simulink model "sampleModel1"  (R2021a)
settings: Solver=VariableStepAuto  StartTime=0.0  StopTime=50  RelTol=1e-3
undefined symbols (not defined in the file): DiscIntNeverNeededParam, magnitude, Newton, Raphson
libraries: simulink x92, pid_lib x10
(part 3 of 5)

== system sampleModel1/cfblk104/cfblk19/cfblk13 ==
  cfblk1 : Inport
  cfblk10 : Inport  Port=2
  cfblk3 : simulink/Discrete/Transfer Fcn Real Zero  ZeroZ=0.75  ICPrevInput=0.0  DoSatur=off
      settings: SourceProductBaseCode=SL
  cfblk4 : Product  Inputs=*
  cfblk5 : Sum  Inputs=+
  cfblk6 : Constant  Value=[-896346582.191985]  SampleTime=1
  cfblk7 : Constant  Value=[-330190841.244627]  SampleTime=1
  cfblk8 : Constant  Value=[644803615.291474]  SampleTime=1
  cfblk9 : Constant  Value=[-669058809.263533]  SampleTime=1
  cfblk2 : Outport
  cfblk11 : Outport  Port=2
  wires:
  cfblk8/1 -> cfblk11/1
  cfblk10/1 -> cfblk5/1
  cfblk9/1 -> cfblk4/1
  cfblk7/1 -> cfblk2/1
  cfblk4/1 -> cfblk3/1

== system sampleModel1/cfblk104/cfblk19/cfblk17 ==
  cfblk1 : Inport
  cfblk15 : Inport  Port=2
  Action Port : ActionPort  ActionPortLabel=if(u1 >= 0)
  cfblk10 : Constant  Value=[-692720338.214887]  SampleTime=1
  cfblk11 : Constant  Value=[-981830203.016373]  SampleTime=1
  cfblk12 : Subsystem
  cfblk13 : Subsystem
  cfblk14 : If  IfExpression=u1 >= 0  SampleTime=1
  cfblk16 : Subsystem  TreatAsAtomicUnit=on
  cfblk17 : Subsystem  TreatAsAtomicUnit=on
  cfblk18 : Delay
  cfblk3 : DiscreteFir
  cfblk4 : UnaryMinus
  cfblk5 : Signum
  cfblk6 : Product  Inputs=**
  cfblk7 : Constant  Value=[115715381.439592]  SampleTime=1
  cfblk8 : Constant  Value=[789801584.459016]  SampleTime=1
  cfblk9 : Constant  Value=[-738286634.708104]  SampleTime=1
  cfblk2 : Outport
  wires:
  cfblk10/1 -> cfblk6/1
  cfblk4/1 -> cfblk17/1(cfblk1)
  cfblk12/1(cfblk2) -> cfblk3/1
  cfblk17/1(cfblk2) -> cfblk2/1
  cfblk11/1 -> cfblk5/1, cfblk12/6(cfblk12)
  cfblk13/1(cfblk2) -> cfblk16/1(cfblk1)
  cfblk12/2(cfblk13) -> cfblk13/1(cfblk1)
  cfblk16/1(cfblk2) -> cfblk17/2(cfblk9)
  cfblk8/1 -> cfblk6/2
  cfblk3/1 -> cfblk16/2(cfblk7)
  cfblk7/1 -> cfblk14/1
  cfblk5/1 -> cfblk12/1(cfblk1)
  cfblk6/1 -> cfblk4/1
  cfblk9/1 -> cfblk12/2(cfblk8)
  cfblk15/1 -> cfblk12/3(cfblk9)
  cfblk1/1 -> cfblk12/4(cfblk10)
  cfblk14/1 -> cfblk16/Action
  cfblk14/2 -> cfblk17/Action
  cfblk13/2(cfblk14) -> cfblk18/1
  cfblk18/1 -> cfblk12/5(cfblk11)

== system sampleModel1/cfblk104/cfblk19/cfblk18 ==
  cfblk1 : Inport
  cfblk8 : Inport  Port=2
  Action Port : ActionPort  ActionPortLabel=else
  cfblk11 : Delay
  cfblk3 : Sqrt  Operator=rSqrt  AlgorithmType=Newton-Raphson  SaturateOnIntegerOverflow=on
  cfblk4 : Sqrt  SaturateOnIntegerOverflow=on
  cfblk5 : ComplexToRealImag
  cfblk6 : Constant  Value=[-692674466.938590]  SampleTime=1
  cfblk7 : Subsystem
  cfblk2 : Outport
  cfblk9 : Outport  Port=2
  cfblk10 : Outport  Port=3
  wires:
  cfblk5/1 -> cfblk10/1
  cfblk4/1 -> cfblk7/1(cfblk1), cfblk9/1
  cfblk8/1 -> cfblk7/2(cfblk9)
  cfblk6/1 -> cfblk4/1
  cfblk1/1 -> cfblk2/1
  cfblk3/1 -> cfblk7/3(cfblk10)
  cfblk7/1(cfblk2) -> cfblk5/1
  cfblk5/2 -> cfblk11/1
  cfblk11/1 -> cfblk3/1

== system sampleModel1/cfblk104/cfblk21/cfblk11 ==
  cfblk1 : Inport
  cfblk13 : Inport  Port=2
  Action Port : ActionPort  ActionPortLabel=if(u1 >= 0)
  cfblk10 : Constant  Value=[-563913250.111774]  SampleTime=1
  cfblk11 : Subsystem
  cfblk12 : Subsystem
  cfblk16 : Delay
  cfblk3 : DiscreteFir
  cfblk4 : Math  Operator=conj  SaturateOnIntegerOverflow=on
  cfblk5 : Gain  Gain=[532058728.474376]
  cfblk6 : Trigonometry
  cfblk7 : simulink/Math Operations/Slider Gain  gain=1  low=0  high=2
  cfblk8 : Constant  Value=[692304688.549677]  SampleTime=1
  cfblk9 : Constant  Value=[191414295.157756]  SampleTime=1
  cfblk2 : Outport
  cfblk14 : Outport  Port=2
  cfblk15 : Outport  Port=3
  wires:
  cfblk9/1 -> cfblk4/1
  cfblk11/1(cfblk2) -> cfblk7/1
  cfblk10/1 -> cfblk14/1
  cfblk3/1 -> cfblk15/1
  cfblk1/1 -> cfblk12/1(cfblk1)
  cfblk4/1 -> cfblk3/1
  cfblk13/1 -> cfblk6/1
  cfblk6/1 -> cfblk5/1
  cfblk8/1 -> cfblk11/1(cfblk1)
  cfblk5/1 -> cfblk2/1
  cfblk12/1(cfblk2) -> cfblk11/2(cfblk10)
  cfblk7/1 -> cfblk16/1
  cfblk16/1 -> cfblk11/3(cfblk11)

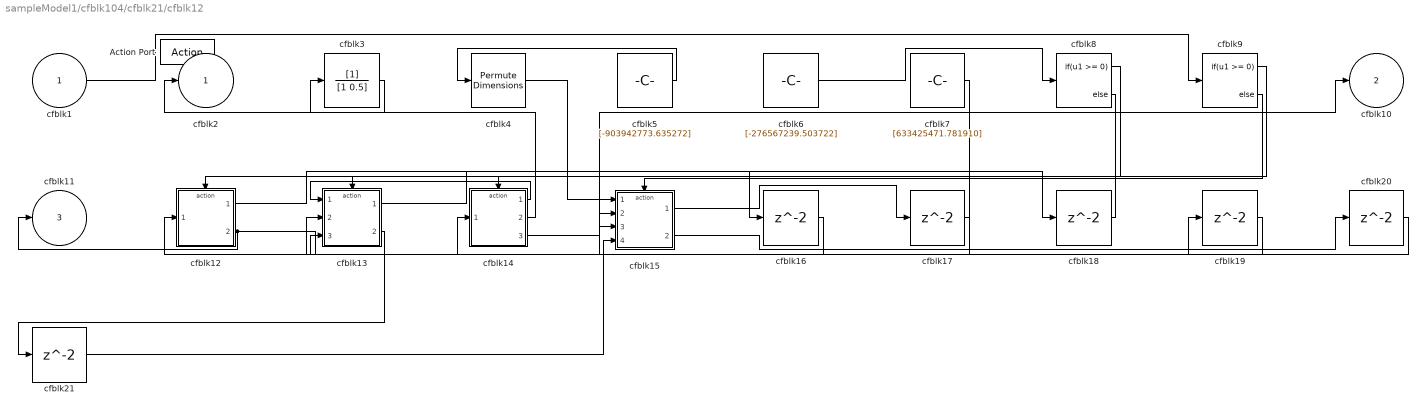
== system sampleModel1/cfblk104/cfblk21/cfblk12 ==
  cfblk1 : Inport
  Action Port : ActionPort  ActionPortLabel=else
  cfblk12 : Subsystem  TreatAsAtomicUnit=on
  cfblk13 : Subsystem  TreatAsAtomicUnit=on
  cfblk14 : Subsystem  TreatAsAtomicUnit=on
  cfblk15 : Subsystem  TreatAsAtomicUnit=on
  cfblk{16..21} (6 alike) : Delay
  cfblk3 : DiscreteFilter
  cfblk4 : PermuteDimensions
  cfblk5 : Constant  Value=[-903942773.635272]  SampleTime=1
  cfblk6 : Constant  Value=[-276567239.503722]  SampleTime=1
  cfblk7 : Constant  Value=[633425471.781910]  SampleTime=1
  cfblk8 : If  IfExpression=u1 >= 0  SampleTime=1
  cfblk9 : If  IfExpression=u1 >= 0  SampleTime=1
  cfblk2 : Outport
  cfblk10 : Outport  Port=2
  cfblk11 : Outport  Port=3
  wires:
  cfblk3/1 -> cfblk2/1
  cfblk5/1 -> cfblk4/1
  cfblk4/1 -> cfblk15/1(cfblk1)
  cfblk7/1 -> cfblk14/1(cfblk1)
  cfblk6/1 -> cfblk8/1
  cfblk12/2(cfblk10) -> cfblk11/1, cfblk19/1
  cfblk1/1 -> cfblk9/1
  cfblk14/1(cfblk2) -> cfblk13/1(cfblk1)
  cfblk14/2(cfblk14) -> cfblk3/1
  cfblk14/3(cfblk15) -> cfblk10/1
  cfblk8/1 -> cfblk12/Action
  cfblk8/2 -> cfblk13/Action
  cfblk9/1 -> cfblk14/Action
  cfblk9/2 -> cfblk15/Action
  cfblk13/1(cfblk2) -> cfblk16/1
  cfblk16/1 -> cfblk15/3(cfblk14)
  cfblk15/1(cfblk2) -> cfblk17/1
  cfblk17/1 -> cfblk12/1(cfblk1)
  cfblk12/1(cfblk2) -> cfblk18/1
  cfblk18/1 -> cfblk15/2(cfblk13)
  cfblk19/1 -> cfblk13/3(cfblk7)
  cfblk15/2(cfblk16) -> cfblk20/1
  cfblk20/1 -> cfblk13/2(cfblk6)
  cfblk13/2(cfblk8) -> cfblk21/1
  cfblk21/1 -> cfblk15/4(cfblk15)

== system sampleModel1/cfblk105/cfblk6/cfblk10 ==
  cfblk1 : Inport
  cfblk12 : Inport  Port=2
  Action Port : ActionPort  ActionPortLabel=else
  cfblk10 : Subsystem
  cfblk11 : If  IfExpression=u1 >= 0  SampleTime=1
  cfblk14 : Subsystem  TreatAsAtomicUnit=on
  cfblk15 : Subsystem  TreatAsAtomicUnit=on
  cfblk16 : Delay
  cfblk17 : Delay
  cfblk18 : Delay
  cfblk3 : ComplexToMagnitudeAngle
  cfblk4 : MinMax  Function=max
  cfblk5 : Trigonometry
  cfblk6 : Product
  cfblk7 : Constant  Value=[986074348.650515]  SampleTime=1
  cfblk8 : Constant  Value=[-373705013.156286]  SampleTime=1
  cfblk9 : Constant  Value=[204800515.931455]  SampleTime=1
  cfblk2 : Outport
  cfblk13 : Outport  Port=2
  wires:
  cfblk6/1 -> cfblk5/1
  cfblk5/1 -> cfblk15/1(cfblk1)
  cfblk9/1 -> cfblk6/1
  cfblk3/1 -> cfblk2/1
  cfblk10/1(cfblk2) -> cfblk13/1
  cfblk14/1(cfblk2) -> cfblk4/1
  cfblk8/1 -> cfblk10/1(cfblk1)
  cfblk10/2(cfblk10) -> cfblk3/1
  cfblk7/1 -> cfblk6/2
  cfblk12/1 -> cfblk14/1(cfblk1)
  cfblk14/2(cfblk15) -> cfblk10/2(cfblk9)
  cfblk14/3(cfblk16) -> cfblk15/2(cfblk9)
  cfblk1/1 -> cfblk14/4(cfblk14)
  cfblk11/1 -> cfblk14/Action
  cfblk11/2 -> cfblk15/Action
  cfblk4/1 -> cfblk16/1
  cfblk16/1 -> cfblk14/2(cfblk12)
  cfblk3/2 -> cfblk17/1
  cfblk17/1 -> cfblk11/1
  cfblk15/1(cfblk2) -> cfblk18/1
  cfblk18/1 -> cfblk14/3(cfblk13)

== system sampleModel1/cfblk105/cfblk6/cfblk9 ==
  cfblk1 : Inport
  cfblk8 : Inport  Port=2
  Action Port : ActionPort  ActionPortLabel=if(u1 >= 0)
  cfblk3 : MinMax  Function=max  Inputs=2
  cfblk4 : simulink/Math Operations/Slider Gain  gain=1  low=0  high=2
  cfblk5 : Polyval  Coefs=[ +2.081618890e-019, -1.441693666e-014, +4.719686976e-010, -8.536869453e-006, +1.621573104e-001, -8.087801117e+001 ]
  cfblk6 : Product  Inputs=**
  cfblk7 : Constant  Value=[-112981505.131855]  SampleTime=1
  cfblk2 : Outport
  wires:
  cfblk5/1 -> cfblk2/1
  cfblk1/1 -> cfblk6/1
  cfblk4/1 -> cfblk3/1
  cfblk3/1 -> cfblk5/1
  cfblk8/1 -> cfblk3/2
  cfblk7/1 -> cfblk6/2
  cfblk6/1 -> cfblk4/1

== system sampleModel1/cfblk108/cfblk9/cfblk7 ==
  cfblk1 : Inport
  cfblk11 : Delay
  cfblk3 : simulink/Discrete/Tapped Delay  vinit=0.0  samptime=-1  NumDelays=1  DelayOrder=Oldest  includeCurrent=off
  cfblk4 : Sum  Inputs=-+
  cfblk5 : Assignment  DiagnosticForDimensions=Warning  IndexOptions=Index vector (dialog)  Indices=1  OutputSizes=1
  cfblk6 : Trigonometry
  cfblk7 : Constant  Value=[85798913.173892]  SampleTime=1
  cfblk8 : Constant  Value=[43764762.818563]  SampleTime=1
  cfblk9 : Constant  Value=[-705776039.354427]  SampleTime=1
  cfblk2 : Outport
  cfblk10 : Outport  Port=2
  wires:
  cfblk7/1 -> cfblk3/1
  cfblk1/1 -> cfblk2/1
  cfblk3/1 -> cfblk5/1
  cfblk9/1 -> cfblk4/2
  cfblk4/1 -> cfblk6/1
  cfblk8/1 -> cfblk5/2
  cfblk5/1 -> cfblk10/1
  cfblk6/1 -> cfblk11/1
  cfblk11/1 -> cfblk4/1

== system sampleModel1/cfblk109/cfblk10/cfblk12 ==
  cfblk1 : Inport
  cfblk10 : Constant  Value=[-373395610.327149]  SampleTime=1
  cfblk11 : Constant  Value=[680026808.036741]  SampleTime=1
  cfblk12 : Delay
  cfblk3 : Sqrt  SaturateOnIntegerOverflow=on
  cfblk4 : Product  Inputs=**
  cfblk5 : Sum  Inputs=+
  cfblk6 : Sin  TimeSource=Use external signal  SampleTime=0
  cfblk7 : Product  Inputs=*
  cfblk8 : UnaryMinus
  cfblk9 : Constant  Value=[715526573.691271]  SampleTime=1
  cfblk2 : Outport
  wires:
  cfblk9/1 -> cfblk2/1
  cfblk4/1 -> cfblk5/1
  cfblk1/1 -> cfblk7/1
  cfblk11/1 -> cfblk6/1
  cfblk8/1 -> cfblk3/1
  cfblk7/1 -> cfblk4/2
  cfblk10/1 -> cfblk8/1
  cfblk5/1 -> cfblk12/1
  cfblk12/1 -> cfblk4/1

== system sampleModel1/cfblk111/cfblk11/cfblk11 ==
  cfblk1 : Inport
  cfblk10 : Inport  Port=2
  cfblk11 : Inport  Port=3
  cfblk12 : Inport  Port=4
  cfblk13 : Inport  Port=5
  cfblk14 : Inport  Port=6
  cfblk15 : Inport  Port=7
  Action Port : ActionPort  ActionPortLabel=if(u1 >= 0)
  cfblk3 : Polyval  Coefs=[ +2.081618890e-019, -1.441693666e-014, +4.719686976e-010, -8.536869453e-006, +1.621573104e-001, -8.087801117e+001 ]
  cfblk4 : Sum  Inputs=-+
  cfblk5 : Constant  Value=[354998664.714576]  SampleTime=1
  cfblk6 : Constant  Value=[363687729.474733]  SampleTime=1
  cfblk7 : Constant  Value=[-525316542.977628]  SampleTime=1
  cfblk8 : Constant  Value=[872838530.440429]  SampleTime=1
  cfblk9 : Subsystem
  cfblk2 : Outport
  cfblk16 : Outport  Port=2
  wires:
  cfblk1/1 -> cfblk4/1
  cfblk9/1(cfblk2) -> cfblk2/1
  cfblk14/1 -> cfblk16/1
  cfblk15/1 -> cfblk9/1(cfblk1)
  cfblk6/1 -> cfblk4/2
  cfblk4/1 -> cfblk9/2(cfblk9)
  cfblk13/1 -> cfblk3/1

== system sampleModel1/cfblk111/cfblk11/cfblk12 ==
  cfblk1 : Inport
  cfblk10 : Inport  Port=2
  cfblk11 : Inport  Port=3
  Action Port : ActionPort  ActionPortLabel=else
  cfblk12 : Subsystem  TreatAsAtomicUnit=on
  cfblk13 : Subsystem  TreatAsAtomicUnit=on
  cfblk14 : Subsystem  TreatAsAtomicUnit=on
  cfblk15 : Subsystem  TreatAsAtomicUnit=on
  cfblk16 : Delay
  cfblk17 : Delay
  cfblk3 : Delay  ShowEnablePort=on
      settings: InputPortMap=u0,e6
  cfblk4 : DotProduct  InputSameDT=on  OutDataTypeStr=Inherit: Inherit via internal rule
  cfblk5 : Sin  TimeSource=Use external signal  SampleTime=0
  cfblk6 : Constant  Value=[-311564060.448794]  SampleTime=1
  cfblk7 : Constant  Value=[687231696.465747]  SampleTime=1
  cfblk8 : If  IfExpression=u1 >= 0  SampleTime=1
  cfblk9 : If  IfExpression=u1 >= 0  SampleTime=1
  cfblk2 : Outport
  wires:
  cfblk6/1 -> cfblk4/1
  cfblk13/1(cfblk2) -> cfblk9/1
  cfblk11/1 -> cfblk5/1
  cfblk4/1 -> cfblk3/1
  cfblk10/1 -> cfblk4/2
  cfblk5/1 -> cfblk3/2
  cfblk12/1(cfblk2) -> cfblk15/1(cfblk1)
  cfblk12/2(cfblk12) -> cfblk15/2(cfblk8)
  cfblk1/1 -> cfblk8/1
  cfblk12/3(cfblk13) -> cfblk13/1(cfblk1)
  cfblk13/2(cfblk15) -> cfblk14/1(cfblk1)
  cfblk7/1 -> cfblk14/2(cfblk9)
  cfblk15/2(cfblk11) -> cfblk2/1
  cfblk14/2(cfblk10) -> cfblk15/3(cfblk9)
  cfblk14/3(cfblk11) -> cfblk15/4(cfblk10)
  cfblk12/4(cfblk14) -> cfblk13/2(cfblk13)
  cfblk3/1 -> cfblk13/3(cfblk14)
  cfblk8/1 -> cfblk12/Action
  cfblk8/2 -> cfblk13/Action
  cfblk9/1 -> cfblk14/Action
  cfblk9/2 -> cfblk15/Action
  cfblk15/1(cfblk2) -> cfblk16/1
  cfblk16/1 -> cfblk12/2(cfblk11)
  cfblk14/1(cfblk2) -> cfblk17/1
  cfblk17/1 -> cfblk12/1(cfblk1)

== system sampleModel1/cfblk111/cfblk11/cfblk5 ==
  cfblk1 : Inport
  cfblk12 : Inport  Port=2
  cfblk10 : Constant  Value=[-453291268.783303]  SampleTime=1
  cfblk11 : Constant  Value=[556035112.715205]  SampleTime=1
  cfblk16 : Delay
  cfblk3 : Abs
  cfblk4 : Sum  Inputs=+
  cfblk5 : PermuteDimensions
  cfblk6 : UnaryMinus
  cfblk7 : Rounding
  cfblk8 : Sin  TimeSource=Use external signal  SampleTime=0
  cfblk9 : Math  Operator=pow  SaturateOnIntegerOverflow=on
  cfblk2 : Outport
  cfblk13 : Outport  Port=2
  cfblk14 : Outport  Port=3
  cfblk15 : Outport  Port=4
  wires:
  cfblk5/1 -> cfblk4/1
  cfblk10/1 -> cfblk9/1
  cfblk1/1 -> cfblk14/1
  cfblk6/1 -> cfblk7/1
  cfblk11/1 -> cfblk2/1
  cfblk9/1 -> cfblk8/1
  cfblk3/1 -> cfblk9/2
  cfblk12/1 -> cfblk6/1, cfblk5/1
  cfblk4/1 -> cfblk15/1
  cfblk7/1 -> cfblk13/1
  cfblk8/1 -> cfblk16/1
  cfblk16/1 -> cfblk3/1

== system sampleModel1/cfblk111/cfblk11/cfblk6 ==
  cfblk1 : Inport
  cfblk7 : Inport  Port=2
  cfblk10 : Delay
  cfblk11 : Delay
  cfblk12 : Delay
  cfblk3 : Sqrt  Operator=rSqrt  AlgorithmType=Newton-Raphson  SaturateOnIntegerOverflow=on
  cfblk4 : Sqrt  Operator=rSqrt  AlgorithmType=Newton-Raphson  SaturateOnIntegerOverflow=on
  cfblk5 : Constant  Value=[-800399417.445094]  SampleTime=1
  cfblk6 : If  IfExpression=u1 >= 0  SampleTime=1
  cfblk8 : Subsystem  TreatAsAtomicUnit=on
  cfblk9 : Subsystem  TreatAsAtomicUnit=on
  cfblk2 : Outport
  wires:
  cfblk1/1 -> cfblk6/1, cfblk9/2(cfblk9)
  cfblk8/1(cfblk2) -> cfblk4/1
  cfblk5/1 -> cfblk8/1(cfblk1)
  cfblk7/1 -> cfblk9/1(cfblk1), cfblk9/4(cfblk11)
  cfblk9/1(cfblk2) -> cfblk3/1
  cfblk3/1 -> cfblk2/1
  cfblk4/1 -> cfblk10/1, cfblk11/1, cfblk12/1
  cfblk6/1 -> cfblk8/Action
  cfblk6/2 -> cfblk9/Action
  cfblk10/1 -> cfblk8/2(cfblk8)
  cfblk11/1 -> cfblk9/3(cfblk10)
  cfblk12/1 -> cfblk9/5(cfblk12)

== system sampleModel1/cfblk111/cfblk11/cfblk7 ==
  cfblk1 : Inport
  cfblk14 : Inport  Port=2
  cfblk10 : Constant  Value=[751520434.957139]  SampleTime=1
  cfblk11 : Constant  Value=[-289698849.543749]  SampleTime=1
  cfblk12 : Subsystem
  cfblk13 : Subsystem
  cfblk3 : Assignment  DiagnosticForDimensions=Warning  IndexOptions=Index vector (dialog)  Indices=1  OutputSizes=1
  cfblk4 : Gain  Gain=[981665956.082482]
  cfblk5 : Math  SaturateOnIntegerOverflow=on
  cfblk6 : Product  Inputs=*
  cfblk7 : Constant  Value=[419064031.236258]  SampleTime=1
  cfblk8 : Constant  Value=[731658762.226406]  SampleTime=1
  cfblk9 : Constant  Value=[910550402.340456]  SampleTime=1
  cfblk2 : Outport
  cfblk15 : Outport  Port=2
  cfblk16 : Outport  Port=3
  cfblk17 : Outport  Port=4
  wires:
  cfblk9/1 -> cfblk3/1, cfblk12/5(cfblk16)
  cfblk13/1(cfblk2) -> cfblk3/2, cfblk12/4(cfblk15)
  cfblk8/1 -> cfblk15/1
  cfblk7/1 -> cfblk6/1
  cfblk14/1 -> cfblk17/1
  cfblk6/1 -> cfblk5/1
  cfblk10/1 -> cfblk16/1
  cfblk5/1 -> cfblk13/1(cfblk1), cfblk13/2(cfblk12), cfblk13/3(cfblk13)
  cfblk1/1 -> cfblk4/1
  cfblk3/1 -> cfblk12/1(cfblk1)
  cfblk12/1(cfblk2) -> cfblk2/1
  cfblk11/1 -> cfblk12/2(cfblk13)
  cfblk4/1 -> cfblk12/3(cfblk14)

== system sampleModel1/cfblk112/cfblk11/cfblk13 ==
  cfblk1 : Inport
  cfblk13 : Inport  Port=2
  Action Port : ActionPort  ActionPortLabel=if(u1 >= 0)
  cfblk10 : simulink/Math Operations/MinMax Running Resettable  Function=min  vinit=0.0
  cfblk11 : ComplexToRealImag
  cfblk12 : If  IfExpression=u1 >= 0  SampleTime=1
  cfblk15 : Subsystem  TreatAsAtomicUnit=on
  cfblk16 : Subsystem  TreatAsAtomicUnit=on
  cfblk17 : Delay
  cfblk18 : Delay
  cfblk3 : simulink/Discrete/Transfer Fcn Real Zero  ZeroZ=0.75  ICPrevInput=0.0  DoSatur=off
      settings: SourceProductBaseCode=SL
  cfblk4 : Delay  DelayLengthSource=Input port
      settings: InputPortMap=u0,p1
  cfblk5 : Delay  DelayLengthSource=Input port
      settings: InputPortMap=u0,p1
  cfblk6 : DiscreteFilter
  cfblk7 : Gain  Gain=[-908813729.133626]
  cfblk8 : ComplexToRealImag
  cfblk9 : Sin  TimeSource=Use external signal  SampleTime=0
  cfblk2 : Outport
  cfblk14 : Outport  Port=2
  wires:
  cfblk10/1 -> cfblk14/1
  cfblk5/1 -> cfblk4/1
  cfblk1/1 -> cfblk7/1
  cfblk16/1(cfblk2) -> cfblk5/1
  cfblk9/1 -> cfblk5/2
  cfblk16/2(cfblk9) -> cfblk10/1
  cfblk11/1 -> cfblk8/1
  cfblk3/1 -> cfblk4/2, cfblk15/4(cfblk13)
  cfblk13/1 -> cfblk11/1
  cfblk8/1 -> cfblk6/1
  cfblk11/2 -> cfblk9/1, cfblk15/5(cfblk14)
  cfblk8/2 -> cfblk10/2, cfblk16/2(cfblk8)
  cfblk7/1 -> cfblk15/1(cfblk1), cfblk15/2(cfblk11), cfblk15/3(cfblk12)
  cfblk6/1 -> cfblk3/1
  cfblk15/1(cfblk2) -> cfblk2/1
  cfblk12/1 -> cfblk15/Action
  cfblk12/2 -> cfblk16/Action
  cfblk15/2(cfblk15) -> cfblk17/1
  cfblk17/1 -> cfblk12/1
  cfblk4/1 -> cfblk18/1
  cfblk18/1 -> cfblk16/1(cfblk1)

== system sampleModel1/cfblk112/cfblk11/cfblk14 ==
  cfblk1 : Inport
  cfblk11 : Inport  Port=2
  cfblk12 : Inport  Port=3
  Action Port : ActionPort  ActionPortLabel=else
  cfblk10 : If  IfExpression=u1 >= 0  SampleTime=1
  cfblk14 : Subsystem  TreatAsAtomicUnit=on
  cfblk15 : Subsystem  TreatAsAtomicUnit=on
  cfblk16 : Delay
  cfblk3 : Gain  Gain=[-812393884.849246]
  cfblk4 : Assignment  DiagnosticForDimensions=Warning  IndexOptions=Index vector (dialog)  Indices=1  OutputSizes=1
  cfblk5 : Math  Operator=rem  SaturateOnIntegerOverflow=on
  cfblk6 : PermuteDimensions
  cfblk7 : Constant  Value=[824090888.558019]  SampleTime=1
  cfblk8 : Constant  Value=[39901777.410130]  SampleTime=1
  cfblk9 : Constant  Value=[370298075.305909]  SampleTime=1
  cfblk2 : Outport
  cfblk13 : Outport  Port=2
  wires:
  cfblk5/1 -> cfblk4/1
  cfblk11/1 -> cfblk6/1
  cfblk8/1 -> cfblk14/1(cfblk1)
  cfblk14/1(cfblk2) -> cfblk2/1
  cfblk12/1 -> cfblk4/2
  cfblk7/1 -> cfblk13/1
  cfblk1/1 -> cfblk5/1
  cfblk6/1 -> cfblk15/1(cfblk1)
  cfblk4/1 -> cfblk3/1
  cfblk3/1 -> cfblk10/1
  cfblk10/1 -> cfblk14/Action
  cfblk10/2 -> cfblk15/Action
  cfblk15/1(cfblk2) -> cfblk16/1
  cfblk16/1 -> cfblk5/2

== system sampleModel1/cfblk112/cfblk12/cfblk8 ==
  cfblk1 : Inport
  cfblk10 : Constant  Value=[706184991.822761]  SampleTime=1
  cfblk11 : Constant  Value=[128369333.683658]  SampleTime=1
  cfblk12 : Constant  Value=[-116794995.497943]  SampleTime=1
  cfblk13 : Constant  Value=[-479914018.681933]  SampleTime=1
  cfblk16 : Delay
  cfblk3 : simulink/Discrete/Tapped Delay  vinit=0.0  samptime=-1  NumDelays=1  DelayOrder=Oldest  includeCurrent=off
  cfblk4 : Signum
  cfblk5 : Sqrt  SaturateOnIntegerOverflow=on
  cfblk6 : ComplexToRealImag
  cfblk7 : Gain  Gain=[906531353.405531]
  cfblk8 : Sum  Inputs=+-
  cfblk9 : Constant  Value=[445096090.367817]  SampleTime=1
  cfblk2 : Outport
  cfblk14 : Outport  Port=2
  cfblk15 : Outport  Port=3
  wires:
  cfblk13/1 -> cfblk15/1
  cfblk12/1 -> cfblk8/1
  cfblk3/1 -> cfblk5/1
  cfblk9/1 -> cfblk6/1
  cfblk11/1 -> cfblk8/2
  cfblk6/1 -> cfblk7/1
  cfblk6/2 -> cfblk14/1
  cfblk10/1 -> cfblk2/1
  cfblk1/1 -> cfblk4/1
  cfblk5/1 -> cfblk16/1
  cfblk16/1 -> cfblk3/1

== system sampleModel1/cfblk114/cfblk11/cfblk12 ==
  cfblk1 : Inport
  cfblk10 : Inport  Port=2
  cfblk11 : Inport  Port=3
  cfblk12 : Inport  Port=4
  cfblk13 : Inport  Port=5
  cfblk14 : Inport  Port=6
  cfblk3 : Sum  Inputs=+-
  cfblk4 : Abs
  cfblk5 : Sin  TimeSource=Use external signal  SampleTime=0
  cfblk6 : Squeeze
  cfblk7 : Bias  Bias=[-305103186.947408]
  cfblk8 : Polyval  Coefs=[ +2.081618890e-019, -1.441693666e-014, +4.719686976e-010, -8.536869453e-006, +1.621573104e-001, -8.087801117e+001 ]
  cfblk9 : Constant  Value=[547781997.778619]  SampleTime=1
  cfblk2 : Outport
  cfblk15 : Outport  Port=2
  cfblk16 : Outport  Port=3
  wires:
  cfblk4/1 -> cfblk15/1
  cfblk14/1 -> cfblk8/1
  cfblk1/1 -> cfblk3/1
  cfblk3/1 -> cfblk5/1
  cfblk13/1 -> cfblk7/1
  cfblk7/1 -> cfblk6/1
  cfblk12/1 -> cfblk4/1
  cfblk9/1 -> cfblk16/1
  cfblk11/1 -> cfblk3/2
  cfblk5/1 -> cfblk2/1

== system sampleModel1/cfblk115/cfblk14/cfblk13 ==
  cfblk1 : Inport
  Action Port : ActionPort  ActionPortLabel=if(u1 >= 0)
  cfblk3 : Reshape
  cfblk4 : Constant  Value=[-939740005.451525]  SampleTime=1
  cfblk5 : Constant  Value=[676322263.453556]  SampleTime=1
  cfblk6 : Constant  Value=[-125315593.883521]  SampleTime=1
  cfblk7 : Constant  Value=[162754948.038243]  SampleTime=1
  cfblk2 : Outport
  cfblk8 : Outport  Port=2
  wires:
  cfblk1/1 -> cfblk2/1
  cfblk6/1 -> cfblk3/1
  cfblk5/1 -> cfblk8/1

== system sampleModel1/cfblk115/cfblk14/cfblk14 ==
  cfblk1 : Inport
  cfblk11 : Inport  Port=2
  Action Port : ActionPort  ActionPortLabel=else
  cfblk10 : Subsystem
  cfblk13 : Delay
  cfblk14 : Delay
  cfblk15 : Delay
  cfblk3 : UnaryMinus
  cfblk4 : Product  Inputs=**
  cfblk5 : Product  Inputs=**
  cfblk6 : Constant  Value=[-206894305.033694]  SampleTime=1
  cfblk7 : Subsystem
  cfblk8 : Subsystem
  cfblk9 : Subsystem
  cfblk2 : Outport
  cfblk12 : Outport  Port=2
  wires:
  cfblk11/1 -> cfblk3/1, cfblk9/5(cfblk13)
  cfblk8/1(cfblk2) -> cfblk9/1(cfblk1)
  cfblk7/1(cfblk2) -> cfblk9/2(cfblk10)
  cfblk3/1 -> cfblk8/1(cfblk1), cfblk12/1
  cfblk6/1 -> cfblk7/1(cfblk1), cfblk4/1
  cfblk10/1(cfblk2) -> cfblk7/2(cfblk9)
  cfblk9/1(cfblk2) -> cfblk5/1, cfblk4/2, cfblk5/2
  cfblk1/1 -> cfblk10/2(cfblk12), cfblk7/4(cfblk11)
  cfblk5/1 -> cfblk13/1, cfblk14/1
  cfblk10/2(cfblk14) -> cfblk7/3(cfblk10)
  cfblk8/2(cfblk9) -> cfblk2/1, cfblk10/3(cfblk13)
  cfblk13/1 -> cfblk9/3(cfblk11)
  cfblk14/1 -> cfblk9/4(cfblk12)
  cfblk4/1 -> cfblk15/1
  cfblk15/1 -> cfblk10/1(cfblk1)

== system sampleModel1/cfblk115/cfblk14/cfblk7 ==
  cfblk1 : Inport
  cfblk10 : Inport  Port=2
  cfblk11 : Inport  Port=3
  cfblk13 : Delay
  cfblk3 : DiscreteTransferFcn
  cfblk4 : Signum
  cfblk5 : Math  Operator=rem  SaturateOnIntegerOverflow=on
  cfblk6 : Product
  cfblk7 : Constant  Value=[190585896.689464]  SampleTime=1
  cfblk8 : Constant  Value=[552798510.555626]  SampleTime=1
  cfblk9 : Constant  Value=[-361012719.051875]  SampleTime=1
  cfblk2 : Outport
  cfblk12 : Outport  Port=2
  wires:
  cfblk8/1 -> cfblk5/1
  cfblk10/1 -> cfblk2/1
  cfblk9/1 -> cfblk3/1
  cfblk4/1 -> cfblk5/2
  cfblk1/1 -> cfblk12/1
  cfblk11/1 -> cfblk6/1
  cfblk3/1 -> cfblk6/2
  cfblk5/1 -> cfblk13/1
  cfblk13/1 -> cfblk4/1

== system sampleModel1/cfblk115/cfblk14/cfblk8 ==
  cfblk1 : Inport
  cfblk12 : Inport  Port=2
  cfblk10 : Constant  Value=[-187166220.545487]  SampleTime=1
  cfblk11 : Constant  Value=[942070970.818746]  SampleTime=1
  cfblk3 : DiscreteTransferFcn
  cfblk4 : Product
  cfblk5 : Reshape
  cfblk6 : Gain  Gain=[466025011.049631]
  cfblk7 : Gain  Gain=[-920602959.198884]
  cfblk8 : Sqrt  Operator=rSqrt  AlgorithmType=Newton-Raphson  SaturateOnIntegerOverflow=on
  cfblk9 : ComplexToMagnitudeAngle
  cfblk2 : Outport
  cfblk13 : Outport  Port=2
  cfblk14 : Outport  Port=3
  wires:
  cfblk10/1 -> cfblk2/1
  cfblk6/1 -> cfblk8/1
  cfblk4/1 -> cfblk7/1
  cfblk5/1 -> cfblk13/1
  cfblk7/1 -> cfblk14/1
  cfblk11/1 -> cfblk6/1
  cfblk8/1 -> cfblk3/1
  cfblk3/1 -> cfblk9/1
  cfblk9/1 -> cfblk4/1
  cfblk12/1 -> cfblk5/1
  cfblk9/2 -> cfblk4/2

== system sampleModel1/cfblk115/cfblk14/cfblk9 ==
  cfblk1 : Inport
  cfblk12 : Inport  Port=2
  cfblk13 : Inport  Port=3
  cfblk10 : Constant  Value=[-911867555.179792]  SampleTime=1
  cfblk11 : Subsystem
  cfblk3 : Sum  Inputs=|++
  cfblk4 : Polyval  Coefs=[ +2.081618890e-019, -1.441693666e-014, +4.719686976e-010, -8.536869453e-006, +1.621573104e-001, -8.087801117e+001 ]
  cfblk5 : Gain  Gain=[922438024.821965]
  cfblk6 : ComplexToRealImag
  cfblk7 : Constant  Value=[512522951.419713]  SampleTime=1
  cfblk8 : Constant  Value=[342533298.063960]  SampleTime=1
  cfblk9 : Constant  Value=[-420316083.713807]  SampleTime=1
  cfblk2 : Outport
  cfblk14 : Outport  Port=2
  cfblk15 : Outport  Port=3
  wires:
  cfblk7/1 -> cfblk4/1
  cfblk9/1 -> cfblk2/1
  cfblk5/1 -> cfblk11/1(cfblk1)
  cfblk8/1 -> cfblk6/1
  cfblk3/1 -> cfblk5/1
  cfblk1/1 -> cfblk3/1
  cfblk10/1 -> cfblk15/1
  cfblk6/1 -> cfblk14/1
  cfblk12/1 -> cfblk3/2
  cfblk6/2 -> cfblk11/2(cfblk7)

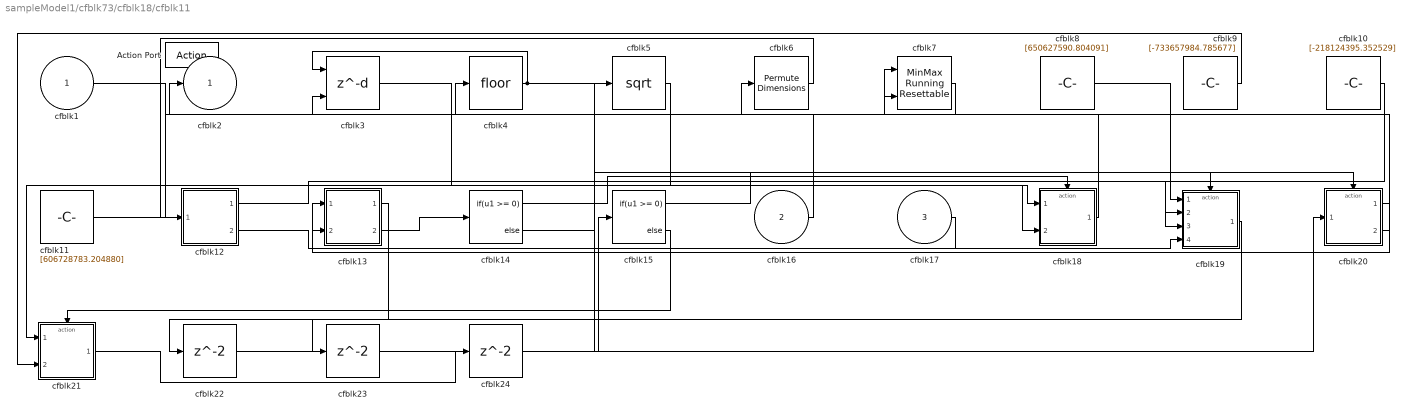
== system sampleModel1/cfblk73/cfblk18/cfblk11 ==
  cfblk1 : Inport
  cfblk16 : Inport  Port=2
  cfblk17 : Inport  Port=3
  Action Port : ActionPort  ActionPortLabel=if(u1 >= 0)
  cfblk10 : Constant  Value=[-218124395.352529]  SampleTime=1
  cfblk11 : Constant  Value=[606728783.204880]  SampleTime=1
  cfblk12 : Subsystem
  cfblk13 : Subsystem
  cfblk14 : If  IfExpression=u1 >= 0  SampleTime=1
  cfblk15 : If  IfExpression=u1 >= 0  SampleTime=1
  cfblk18 : Subsystem  TreatAsAtomicUnit=on
  cfblk19 : Subsystem  TreatAsAtomicUnit=on
  cfblk20 : Subsystem  TreatAsAtomicUnit=on
  cfblk21 : Subsystem  TreatAsAtomicUnit=on
  cfblk22 : Delay
  cfblk23 : Delay
  cfblk24 : Delay
  cfblk3 : Delay  DelayLengthSource=Input port
      settings: InputPortMap=u0,p1
  cfblk4 : Rounding
  cfblk5 : Sqrt  SaturateOnIntegerOverflow=on
  cfblk6 : PermuteDimensions
  cfblk7 : simulink/Math Operations/MinMax Running Resettable  Function=min  vinit=0.0
  cfblk8 : Constant  Value=[650627590.804091]  SampleTime=1
  cfblk9 : Constant  Value=[-733657984.785677]  SampleTime=1
  cfblk2 : Outport
  wires:
  cfblk7/1 -> cfblk2/1
  cfblk6/1 -> cfblk12/1(cfblk1)
  cfblk20/1(cfblk2) -> cfblk13/1(cfblk1)
  cfblk17/1 -> cfblk13/2(cfblk13)
  cfblk18/1(cfblk2) -> cfblk7/1
  cfblk8/1 -> cfblk19/1(cfblk1)
  cfblk16/1 -> cfblk6/1
  cfblk5/1 -> cfblk21/1(cfblk1)
  cfblk10/1 -> cfblk19/2(cfblk13)
  cfblk20/2(cfblk9) -> cfblk4/1
  cfblk9/1 -> cfblk21/2(cfblk8)
  cfblk12/1(cfblk2) -> cfblk19/3(cfblk14)
  cfblk4/1 -> cfblk3/1, cfblk18/2(cfblk10)
  cfblk13/2(cfblk14) -> cfblk14/1
  cfblk12/2(cfblk11) -> cfblk19/4(cfblk15)
  cfblk11/1 -> cfblk7/2
  cfblk1/1 -> cfblk3/2
  cfblk3/1 -> cfblk18/1(cfblk1)
  cfblk14/1 -> cfblk18/Action
  cfblk14/2 -> cfblk19/Action
  cfblk15/1 -> cfblk20/Action
  cfblk15/2 -> cfblk21/Action
  cfblk13/1(cfblk2) -> cfblk22/1
  cfblk22/1 -> cfblk20/1(cfblk1)
  cfblk19/1(cfblk2) -> cfblk23/1
  cfblk23/1 -> cfblk5/1
  cfblk21/1(cfblk2) -> cfblk24/1
  cfblk24/1 -> cfblk15/1

== system sampleModel1/cfblk73/cfblk18/cfblk12 ==
  cfblk1 : Inport
  cfblk6 : Inport  Port=2
  Action Port : ActionPort  ActionPortLabel=else
  cfblk3 : Constant  Value=[630794422.954842]  SampleTime=1
  cfblk4 : Constant  Value=[977823232.159178]  SampleTime=1
  cfblk5 : If  IfExpression=u1 >= 0  SampleTime=1
  cfblk8 : Subsystem  TreatAsAtomicUnit=on
  cfblk9 : Subsystem  TreatAsAtomicUnit=on
  cfblk2 : Outport
  cfblk7 : Outport  Port=2
  wires:
  cfblk4/1 -> cfblk9/1(cfblk1)
  cfblk3/1 -> cfblk8/1(cfblk1), cfblk8/4(cfblk11)
  cfblk1/1 -> cfblk5/1
  cfblk8/1(cfblk2) -> cfblk2/1
  cfblk9/1(cfblk2) -> cfblk7/1
  cfblk6/1 -> cfblk8/2(cfblk9), cfblk8/3(cfblk10)
  cfblk5/1 -> cfblk8/Action
  cfblk5/2 -> cfblk9/Action

== system sampleModel1/cfblk89/cfblk11/cfblk13 ==
  cfblk1 : Inport
  cfblk10 : Inport  Port=2
  Action Port : ActionPort  ActionPortLabel=if(u1 >= 0)
  cfblk3 : DiscreteTransferFcn
  cfblk4 : Bias  Bias=[-984359412.861330]
  cfblk5 : Assignment  DiagnosticForDimensions=Warning  IndexOptions=Index vector (dialog)  Indices=1  OutputSizes=1
  cfblk6 : Constant  Value=[-153781229.671667]  SampleTime=1
  cfblk7 : Constant  Value=[445845049.384049]  SampleTime=1
  cfblk8 : Constant  Value=[-782364123.453909]  SampleTime=1
  cfblk9 : Subsystem
  cfblk2 : Outport
  wires:
  cfblk5/1 -> cfblk3/1
  cfblk6/1 -> cfblk4/1
  cfblk7/1 -> cfblk5/1
  cfblk4/1 -> cfblk9/1(cfblk1)
  cfblk1/1 -> cfblk2/1
  cfblk8/1 -> cfblk5/2

== system sampleModel1/cfblk89/cfblk11/cfblk14 ==
  cfblk1 : Inport
  cfblk6 : Inport  Port=2
  cfblk7 : Inport  Port=3
  cfblk8 : Inport  Port=4
  Action Port : ActionPort  ActionPortLabel=else
  cfblk3 : Sin  TimeSource=Use external signal  SampleTime=0
  cfblk4 : Constant  Value=[-788159166.534469]  SampleTime=1
  cfblk5 : Subsystem
  cfblk2 : Outport
  cfblk9 : Outport  Port=2
  cfblk10 : Outport  Port=3
  wires:
  cfblk6/1 -> cfblk9/1
  cfblk4/1 -> cfblk3/1
  cfblk3/1 -> cfblk10/1
  cfblk8/1 -> cfblk5/1(cfblk1)
  cfblk7/1 -> cfblk5/2(cfblk11)
  cfblk5/1(cfblk2) -> cfblk2/1

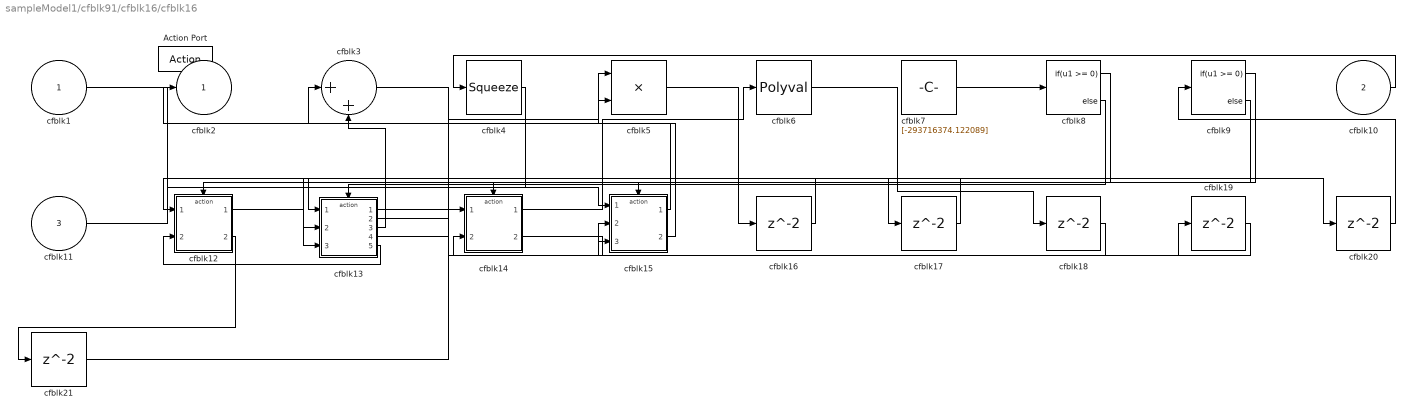
== system sampleModel1/cfblk91/cfblk16/cfblk16 ==
  cfblk1 : Inport
  cfblk10 : Inport  Port=2
  cfblk11 : Inport  Port=3
  Action Port : ActionPort  ActionPortLabel=if(u1 >= 0)
  cfblk12 : Subsystem  TreatAsAtomicUnit=on
  cfblk13 : Subsystem  TreatAsAtomicUnit=on
  cfblk14 : Subsystem  TreatAsAtomicUnit=on
  cfblk15 : Subsystem  TreatAsAtomicUnit=on
  cfblk{16..21} (6 alike) : Delay
  cfblk3 : Sum  Inputs=|++
  cfblk4 : Squeeze
  cfblk5 : Product
  cfblk6 : Polyval  Coefs=[ +2.081618890e-019, -1.441693666e-014, +4.719686976e-010, -8.536869453e-006, +1.621573104e-001, -8.087801117e+001 ]
  cfblk7 : Constant  Value=[-293716374.122089]  SampleTime=1
  cfblk8 : If  IfExpression=u1 >= 0  SampleTime=1
  cfblk9 : If  IfExpression=u1 >= 0  SampleTime=1
  cfblk2 : Outport
  wires:
  cfblk14/1(cfblk2) -> cfblk6/1
  cfblk7/1 -> cfblk8/1
  cfblk13/1(cfblk2) -> cfblk5/1
  cfblk13/2(cfblk14) -> cfblk15/1(cfblk1)
  cfblk1/1 -> cfblk13/2(cfblk12)
  cfblk11/1 -> cfblk5/2
  cfblk15/1(cfblk2) -> cfblk3/1
  cfblk15/2(cfblk14) -> cfblk2/1
  cfblk13/3(cfblk15) -> cfblk3/2
  cfblk4/1 -> cfblk13/3(cfblk13)
  cfblk13/4(cfblk16) -> cfblk15/2(cfblk12)
  cfblk10/1 -> cfblk4/1
  cfblk13/5(cfblk17) -> cfblk12/2(cfblk16)
  cfblk8/1 -> cfblk12/Action
  cfblk8/2 -> cfblk13/Action
  cfblk9/1 -> cfblk14/Action
  cfblk9/2 -> cfblk15/Action
  cfblk5/1 -> cfblk16/1
  cfblk16/1 -> cfblk13/1(cfblk1)
  cfblk3/1 -> cfblk17/1
  cfblk17/1 -> cfblk12/1(cfblk1)
  cfblk6/1 -> cfblk18/1
  cfblk18/1 -> cfblk14/2(cfblk9)
  cfblk14/2(cfblk10) -> cfblk19/1
  cfblk19/1 -> cfblk15/3(cfblk13)
  cfblk12/1(cfblk2) -> cfblk20/1
  cfblk20/1 -> cfblk9/1
  cfblk12/2(cfblk17) -> cfblk21/1
  cfblk21/1 -> cfblk14/1(cfblk1)

== system sampleModel1/cfblk91/cfblk16/cfblk17 ==
  cfblk1 : Inport
  cfblk10 : Inport  Port=2
  cfblk11 : Inport  Port=3
  cfblk12 : Inport  Port=4
  Action Port : ActionPort  ActionPortLabel=else
  cfblk3 : UnitDelay  SampleTime=-1  HasFrameUpgradeWarning=on
  cfblk4 : Assignment  DiagnosticForDimensions=Warning  IndexOptions=Index vector (dialog)  Indices=1  OutputSizes=1
  cfblk5 : Product
  cfblk6 : Product
  cfblk7 : Constant  Value=[171218251.403757]  SampleTime=1
  cfblk8 : Constant  Value=[-834074701.778912]  SampleTime=1
  cfblk9 : Constant  Value=[33958029.412426]  SampleTime=1
  cfblk2 : Outport
  cfblk13 : Outport  Port=2
  wires:
  cfblk8/1 -> cfblk13/1
  cfblk12/1 -> cfblk4/1
  cfblk6/1 -> cfblk5/1
  cfblk7/1 -> cfblk6/1
  cfblk10/1 -> cfblk4/2
  cfblk4/1 -> cfblk3/1
  cfblk11/1 -> cfblk5/2
  cfblk1/1 -> cfblk2/1
  cfblk3/1 -> cfblk6/2

== system sampleModel1/cfblk91/cfblk18/cfblk14 ==
  cfblk1 : Inport
  Action Port : ActionPort  ActionPortLabel=if(u1 >= 0)
  cfblk10 : Subsystem  TreatAsAtomicUnit=on
  cfblk11 : Subsystem  TreatAsAtomicUnit=on
  cfblk3 : DiscreteIntegrator  SampleTime=-1  ICPrevOutput=DiscIntNeverNeededParam  ICPrevScaledInput=DiscIntNeverNeededParam
  cfblk4 : simulink/Math Operations/Slider Gain  gain=1  low=0  high=2
  cfblk5 : simulink/Math Operations/Slider Gain  gain=1  low=0  high=2
  cfblk6 : Constant  Value=[152111802.993114]  SampleTime=1
  cfblk7 : Constant  Value=[291069011.962643]  SampleTime=1
  cfblk8 : Constant  Value=[8795720.185533]  SampleTime=1
  cfblk9 : If  IfExpression=u1 >= 0  SampleTime=1
  cfblk2 : Outport
  wires:
  cfblk6/1 -> cfblk2/1
  cfblk3/1 -> cfblk9/1
  cfblk10/1(cfblk2) -> cfblk11/1(cfblk1)
  cfblk7/1 -> cfblk10/1(cfblk1)
  cfblk8/1 -> cfblk3/1
  cfblk11/1(cfblk2) -> cfblk4/1
  cfblk4/1 -> cfblk5/1
  cfblk9/1 -> cfblk10/Action
  cfblk9/2 -> cfblk11/Action

== system sampleModel1/cfblk91/cfblk18/cfblk15 ==
  cfblk1 : Inport
  cfblk7 : Inport  Port=2
  Action Port : ActionPort  ActionPortLabel=else
  cfblk10 : Subsystem  TreatAsAtomicUnit=on
  cfblk11 : Subsystem  TreatAsAtomicUnit=on
  cfblk12 : Subsystem  TreatAsAtomicUnit=on
  cfblk{13..19} (7 alike) : Delay
  cfblk3 : DotProduct  InputSameDT=on  OutDataTypeStr=Inherit: Inherit via internal rule
  cfblk4 : Squeeze
  cfblk5 : If  IfExpression=u1 >= 0  SampleTime=1
  cfblk6 : If  IfExpression=u1 >= 0  SampleTime=1
  cfblk9 : Subsystem  TreatAsAtomicUnit=on
  cfblk2 : Outport
  cfblk8 : Outport  Port=2
  wires:
  cfblk7/1 -> cfblk10/1(cfblk1)
  cfblk1/1 -> cfblk6/1, cfblk11/4(cfblk12), cfblk5/1, cfblk11/5(cfblk13)
  cfblk3/1 -> cfblk2/1
  cfblk4/1 -> cfblk16/1, cfblk17/1
  cfblk9/1(cfblk2) -> cfblk4/1
  cfblk12/2(cfblk17) -> cfblk15/1, cfblk18/1
  cfblk10/2(cfblk13) -> cfblk8/1
  cfblk10/3(cfblk14) -> cfblk3/2, cfblk19/1
  cfblk11/1(cfblk2) -> cfblk3/1
  cfblk11/2(cfblk14) -> cfblk10/2(cfblk11)
  cfblk11/3(cfblk15) -> cfblk12/2(cfblk15), cfblk12/3(cfblk16)
  cfblk5/1 -> cfblk9/Action
  cfblk5/2 -> cfblk10/Action
  cfblk6/1 -> cfblk11/Action
  cfblk6/2 -> cfblk12/Action
  cfblk10/1(cfblk2) -> cfblk13/1
  cfblk13/1 -> cfblk12/1(cfblk1)
  cfblk12/1(cfblk2) -> cfblk14/1
  cfblk14/1 -> cfblk11/1(cfblk1)
  cfblk15/1 -> cfblk9/2(cfblk7)
  cfblk16/1 -> cfblk9/1(cfblk1)
  cfblk17/1 -> cfblk11/3(cfblk11)
  cfblk18/1 -> cfblk10/3(cfblk12)
  cfblk19/1 -> cfblk11/2(cfblk10)

== system sampleModel1/cfblk92/cfblk17/cfblk11 ==
  cfblk1 : Inport
  cfblk10 : Inport  Port=2
  Action Port : ActionPort  ActionPortLabel=if(u1 >= 0)
  cfblk14 : Subsystem  TreatAsAtomicUnit=on
  cfblk15 : Subsystem  TreatAsAtomicUnit=on
  cfblk16 : Delay
  cfblk3 : Rounding
  cfblk4 : Constant  Value=[-783127144.288970]  SampleTime=1
  cfblk5 : Constant  Value=[236182478.093947]  SampleTime=1
  cfblk6 : Constant  Value=[923929315.610652]  SampleTime=1
  cfblk7 : Subsystem
  cfblk8 : Subsystem
  cfblk9 : If  IfExpression=u1 >= 0  SampleTime=1
  cfblk2 : Outport
  cfblk11 : Outport  Port=2
  cfblk12 : Outport  Port=3
  cfblk13 : Outport  Port=4
  wires:
  cfblk15/1(cfblk2) -> cfblk11/1
  cfblk4/1 -> cfblk7/1(cfblk1), cfblk14/6(cfblk14)
  cfblk1/1 -> cfblk15/1(cfblk1), cfblk14/5(cfblk13)
  cfblk10/1 -> cfblk8/1(cfblk1)
  cfblk7/1(cfblk2) -> cfblk13/1
  cfblk14/1(cfblk2) -> cfblk12/1
  cfblk8/2(cfblk15) -> cfblk2/1
  cfblk7/2(cfblk13) -> cfblk8/2(cfblk12)
  cfblk15/2(cfblk15) -> cfblk14/1(cfblk1)
  cfblk5/1 -> cfblk9/1
  cfblk15/3(cfblk16) -> cfblk14/2(cfblk10)
  cfblk15/4(cfblk17) -> cfblk14/3(cfblk11)
  cfblk3/1 -> cfblk8/3(cfblk13)
  cfblk7/3(cfblk14) -> cfblk8/4(cfblk14)
  cfblk6/1 -> cfblk14/4(cfblk12)
  cfblk9/1 -> cfblk14/Action
  cfblk9/2 -> cfblk15/Action
  cfblk8/1(cfblk2) -> cfblk16/1
  cfblk16/1 -> cfblk3/1

== system sampleModel1/cfblk92/cfblk17/cfblk12 ==
  cfblk1 : Inport
  cfblk10 : Inport  Port=2
  Action Port : ActionPort  ActionPortLabel=else
  cfblk11 : Delay
  cfblk3 : Delay
  cfblk4 : Sum  Inputs=+
  cfblk5 : Bias  Bias=[835760183.997279]
  cfblk6 : Sum  Inputs=+-
  cfblk7 : Sqrt  SaturateOnIntegerOverflow=on
  cfblk8 : Constant  Value=[-725392683.108246]  SampleTime=1
  cfblk9 : Constant  Value=[-190083039.765405]  SampleTime=1
  cfblk2 : Outport
  wires:
  cfblk6/1 -> cfblk3/1
  cfblk5/1 -> cfblk7/1
  cfblk4/1 -> cfblk6/1
  cfblk3/1 -> cfblk2/1
  cfblk8/1 -> cfblk6/2
  cfblk9/1 -> cfblk4/1
  cfblk7/1 -> cfblk11/1
  cfblk11/1 -> cfblk5/1

== system sampleModel1/cfblk92/cfblk18/cfblk10 ==
  cfblk1 : Inport
  cfblk12 : Inport  Port=2
  cfblk13 : Inport  Port=3
  cfblk14 : Inport  Port=4
  cfblk15 : Inport  Port=5
  cfblk16 : Inport  Port=6
  Action Port : ActionPort  ActionPortLabel=else
  cfblk10 : Constant  Value=[799871001.052351]  SampleTime=1
  cfblk11 : Subsystem
  cfblk3 : Delay  DelayLengthSource=Input port
      settings: InputPortMap=u0,p1
  cfblk4 : simulink/Discrete/Tapped Delay  vinit=0.0  samptime=-1  NumDelays=1  DelayOrder=Oldest  includeCurrent=off
  cfblk5 : Delay  ShowEnablePort=on
      settings: InputPortMap=u0,e6
  cfblk6 : Gain  Gain=[631974506.592415]
  cfblk7 : Sum  Inputs=|++
  cfblk8 : Constant  Value=[-803325396.510725]  SampleTime=1
  cfblk9 : Constant  Value=[-944741983.677650]  SampleTime=1
  cfblk2 : Outport
  cfblk17 : Outport  Port=2
  wires:
  cfblk7/1 -> cfblk4/1
  cfblk4/1 -> cfblk5/1
  cfblk13/1 -> cfblk5/2
  cfblk12/1 -> cfblk3/1
  cfblk9/1 -> cfblk6/1
  cfblk3/1 -> cfblk2/1
  cfblk6/1 -> cfblk11/1(cfblk1)
  cfblk16/1 -> cfblk11/2(cfblk6)
  cfblk14/1 -> cfblk11/3(cfblk7)
  cfblk11/1(cfblk2) -> cfblk17/1
  cfblk15/1 -> cfblk7/1
  cfblk5/1 -> cfblk3/2
  cfblk11/2(cfblk8) -> cfblk7/2

== system sampleModel1/cfblk92/cfblk18/cfblk6 ==
  cfblk1 : Inport
  cfblk9 : Inport  Port=2
  cfblk10 : Inport  Port=3
  cfblk11 : Subsystem  TreatAsAtomicUnit=on
  cfblk12 : Subsystem  TreatAsAtomicUnit=on
  cfblk13 : Delay
  cfblk14 : Delay
  cfblk15 : Delay
  cfblk3 : PermuteDimensions
  cfblk4 : Sum  Inputs=--
  cfblk5 : simulink/Math Operations/Slider Gain  gain=1  low=0  high=2
  cfblk6 : Product  Inputs=**
  cfblk7 : Constant  Value=[803547328.095126]  SampleTime=1
  cfblk8 : If  IfExpression=u1 >= 0  SampleTime=1
  cfblk2 : Outport
  wires:
  cfblk7/1 -> cfblk5/1
  cfblk1/1 -> cfblk3/1
  cfblk12/1(cfblk2) -> cfblk2/1
  cfblk12/2(cfblk12) -> cfblk6/1
  cfblk12/3(cfblk13) -> cfblk11/2(cfblk11)
  cfblk3/1 -> cfblk12/1(cfblk1)
  cfblk12/4(cfblk14) -> cfblk6/2
  cfblk5/1 -> cfblk4/1
  cfblk4/1 -> cfblk12/2(cfblk10)
  cfblk10/1 -> cfblk4/2
  cfblk8/1 -> cfblk11/Action
  cfblk8/2 -> cfblk12/Action
  cfblk6/1 -> cfblk13/1
  cfblk13/1 -> cfblk11/1(cfblk1)
  cfblk11/1(cfblk2) -> cfblk14/1
  cfblk14/1 -> cfblk8/1
  cfblk11/2(cfblk12) -> cfblk15/1
  cfblk15/1 -> cfblk12/3(cfblk11)

== system sampleModel1/cfblk92/cfblk18/cfblk9 ==
  cfblk1 : Inport
  cfblk8 : Inport  Port=2
  Action Port : ActionPort  ActionPortLabel=if(u1 >= 0)
  cfblk3 : simulink/Discrete/Transfer Fcn Lead or Lag  PoleZ=0.95  ZeroZ=0.75  ICPrevOutput=0.0  ICPrevInput=0.0  DoSatur=off
      settings: SourceProductBaseCode=SL
  cfblk4 : Delay
  cfblk5 : ComplexToMagnitudeAngle
  cfblk6 : Constant  Value=[759732880.568005]  SampleTime=1
  cfblk7 : Constant  Value=[-294879797.502721]  SampleTime=1
  cfblk2 : Outport
  cfblk9 : Outport  Port=2
  wires:
  cfblk7/1 -> cfblk4/1
  cfblk4/1 -> cfblk5/1
  cfblk6/1 -> cfblk2/1
  cfblk5/1 -> cfblk3/1
  cfblk1/1 -> cfblk9/1

== system sampleModel1/cfblk96/cfblk11/cfblk10 ==
  cfblk1 : Inport
  cfblk3 : simulink/Discrete/Transfer Fcn Lead or Lag  PoleZ=0.95  ZeroZ=0.75  ICPrevOutput=0.0  ICPrevInput=0.0  DoSatur=off
      settings: SourceProductBaseCode=SL
  cfblk4 : DotProduct  InputSameDT=on  OutDataTypeStr=Inherit: Inherit via internal rule
  cfblk5 : Constant  Value=[768845318.187150]  SampleTime=1
  cfblk6 : Constant  Value=[-243703123.835714]  SampleTime=1
  cfblk2 : Outport
  cfblk7 : Outport  Port=2
  wires:
  cfblk6/1 -> cfblk3/1
  cfblk4/1 -> cfblk2/1
  cfblk5/1 -> cfblk7/1
  cfblk1/1 -> cfblk4/1
  cfblk3/1 -> cfblk4/2

== system sampleModel1/cfblk96/cfblk11/cfblk11 ==
  cfblk1 : Inport
  cfblk15 : Inport  Port=2
  cfblk10 : Constant  Value=[-845025036.969157]  SampleTime=1
  cfblk11 : Constant  Value=[-710946186.102976]  SampleTime=1
  cfblk12 : Constant  Value=[244782866.162502]  SampleTime=1
  cfblk13 : Subsystem
  cfblk14 : If  IfExpression=u1 >= 0  SampleTime=1
  cfblk16 : Subsystem  TreatAsAtomicUnit=on
  cfblk17 : Subsystem  TreatAsAtomicUnit=on
  cfblk18 : Delay
  cfblk19 : Delay
  cfblk20 : Delay
  cfblk3 : simulink/Discrete/Transfer Fcn Lead or Lag  PoleZ=0.95  ZeroZ=0.75  ICPrevOutput=0.0  ICPrevInput=0.0  DoSatur=off
      settings: SourceProductBaseCode=SL
  cfblk4 : Signum
  cfblk5 : UnaryMinus
  cfblk6 : Assignment  DiagnosticForDimensions=Warning  IndexOptions=Index vector (dialog)  Indices=1  OutputSizes=1
  cfblk7 : Sum  Inputs=+
  cfblk8 : Product
  cfblk9 : Constant  Value=[229807130.280110]  SampleTime=1
  cfblk2 : Outport
  wires:
  cfblk10/1 -> cfblk2/1
  cfblk8/1 -> cfblk13/1(cfblk1)
  cfblk13/1(cfblk2) -> cfblk3/1
  cfblk15/1 -> cfblk17/1(cfblk1)
  cfblk6/1 -> cfblk5/1
  cfblk11/1 -> cfblk6/1
  cfblk4/1 -> cfblk13/2(cfblk10)
  cfblk12/1 -> cfblk4/1
  cfblk1/1 -> cfblk17/2(cfblk14)
  cfblk17/1(cfblk2) -> cfblk6/2
  cfblk17/2(cfblk15) -> cfblk8/1
  cfblk9/1 -> cfblk7/1
  cfblk16/1(cfblk2) -> cfblk13/3(cfblk11)
  cfblk7/1 -> cfblk8/2
  cfblk14/1 -> cfblk16/Action
  cfblk14/2 -> cfblk17/Action
  cfblk5/1 -> cfblk18/1
  cfblk18/1 -> cfblk16/2(cfblk13)
  cfblk3/1 -> cfblk19/1
  cfblk19/1 -> cfblk14/1
  cfblk13/2(cfblk12) -> cfblk20/1
  cfblk20/1 -> cfblk16/1(cfblk1)

== system sampleModel1/cfblk99/cfblk10/cfblk9 ==
  cfblk1 : Inport
  cfblk8 : Inport  Port=2
  cfblk3 : Sum  Inputs=|++
  cfblk4 : simulink/Math Operations/MinMax Running Resettable  Function=min  vinit=0.0
  cfblk5 : Constant  Value=[214514771.768079]  SampleTime=1
  cfblk6 : Constant  Value=[849544862.366396]  SampleTime=1
  cfblk7 : Constant  Value=[-791000664.204850]  SampleTime=1
  cfblk2 : Outport
  cfblk9 : Outport  Port=2
  cfblk10 : Outport  Port=3
  cfblk11 : Outport  Port=4
  wires:
  cfblk1/1 -> cfblk4/1
  cfblk5/1 -> cfblk3/1
  cfblk7/1 -> cfblk3/2
  cfblk6/1 -> cfblk10/1
  cfblk4/1 -> cfblk9/1, cfblk2/1
  cfblk8/1 -> cfblk11/1
  cfblk3/1 -> cfblk4/2

== system sampleModel1/cfblk99/cfblk9/cfblk12 ==
  cfblk1 : Inport
  cfblk11 : Inport  Port=2
  cfblk12 : Inport  Port=3
  cfblk13 : Inport  Port=4
  Action Port : ActionPort  ActionPortLabel=if(u1 >= 0)
  cfblk10 : If  IfExpression=u1 >= 0  SampleTime=1
  cfblk16 : Subsystem  TreatAsAtomicUnit=on
  cfblk17 : Subsystem  TreatAsAtomicUnit=on
  cfblk18 : Delay
  cfblk3 : Squeeze
  cfblk4 : Trigonometry
  cfblk5 : Rounding
  cfblk6 : Signum
  cfblk7 : Constant  Value=[136707837.339884]  SampleTime=1
  cfblk8 : Constant  Value=[269158969.620844]  SampleTime=1
  cfblk9 : Constant  Value=[-184761110.108189]  SampleTime=1
  cfblk2 : Outport
  cfblk14 : Outport  Port=2
  cfblk15 : Outport  Port=3
  wires:
  cfblk17/1(cfblk2) -> cfblk15/1
  cfblk5/1 -> cfblk6/1
  cfblk4/1 -> cfblk16/1(cfblk1)
  cfblk9/1 -> cfblk3/1
  cfblk12/1 -> cfblk14/1, cfblk17/6(cfblk14)
  cfblk3/1 -> cfblk2/1
  cfblk13/1 -> cfblk5/1, cfblk17/7(cfblk15)
  cfblk7/1 -> cfblk17/1(cfblk1)
  cfblk11/1 -> cfblk4/1
  cfblk6/1 -> cfblk17/2(cfblk10)
  cfblk1/1 -> cfblk16/2(cfblk11), cfblk17/5(cfblk13)
  cfblk8/1 -> cfblk17/3(cfblk11)
  cfblk16/2(cfblk12) -> cfblk17/4(cfblk12)
  cfblk10/1 -> cfblk16/Action
  cfblk10/2 -> cfblk17/Action
  cfblk16/1(cfblk2) -> cfblk18/1
  cfblk18/1 -> cfblk10/1

== system sampleModel1/cfblk99/cfblk9/cfblk13 ==
  cfblk1 : Inport
  Action Port : ActionPort  ActionPortLabel=else
  cfblk10 : Constant  Value=[558979003.687947]  SampleTime=1
  cfblk11 : Subsystem
  cfblk12 : Subsystem
  cfblk13 : If  IfExpression=u1 >= 0  SampleTime=1
  cfblk15 : Subsystem  TreatAsAtomicUnit=on
  cfblk16 : Subsystem  TreatAsAtomicUnit=on
  cfblk17 : Delay
  cfblk18 : Delay
  cfblk3 : pid_lib/PID Controller  Controller=PID  Form=Parallel  TimeDomain=Discrete-time  UseExternalTs=off  SampleTime=-1  IntegratorMethod=Forward Euler  FilterMethod=Forward Euler  ControllerParametersSource=internal  P=1  I=1  D=0  UseFilter=on  N=100  TunerSelectOption=Transfer Function Based (PID Tuner App)  InitialConditionSource=internal  InitialConditionForIntegrator=0  InitialConditionForFilter=0  DifferentiatorICPrevScaledInput=0  ExternalReset=none  TrackingMode=off  Kt=1  LimitOutput=off  SatLimitsSource=internal  UpperSaturationLimit=inf  LowerSaturationLimit=-inf  LinearizeAsGain=off  AntiWindupMode=none  Kb=1  POutMin=[]  POutMax=[]  IOutMin=[]  IOutMax=[]  DOutMin=[]  DOutMax=[]  NOutMin=[]  NOutMax=[]  SumOutMin=[]  SumOutMax=[]  SaturationOutMin=[]  SaturationOutMax=[]  PParamMin=[]  PParamMax=[]  IParamMin=[]  IParamMax=[]  DParamMin=[]  DParamMax=[]  NParamMin=[]  NParamMax=[]  KbParamMin=[]  KbParamMax=[]  KtParamMin=[]  KtParamMax=[]  KbOutMin=[]  KbOutMax=[]  KtOutMin=[]  KtOutMax=[]  IntegratorOutMin=[]  IntegratorOutMax=[]  FilterOutMin=[]  FilterOutMax=[]  SumI1OutMin=[]  SumI1OutMax=[]  SumI2OutMin=[]  SumI2OutMax=[]  SumI3OutMin=[]  SumI3OutMax=[]  SumI4OutMin=[]  SumI4OutMax=[]  SumDOutMin=[]  SumDOutMax=[]  DifferentiatorOutMin=[]  DifferentiatorOutMax=[]  FilterDiffOutCoefMin=[]  FilterDiffOutCoefMax=[]  ReciprocalOutMin=[]  ReciprocalOutMax=[]  SumDenOutMin=[]  SumDenOutMax=[]  SumNumOutMin=[]  SumNumOutMax=[]  DivideOutMin=[]  DivideOutMax=[]  UdiffTsProdOutMin=[]  UdiffTsProdOutMax=[]  NTsProdOutMin=[]  NTsProdOutMax=[]  UintegralTsProdOutMin=[]  UintegralTsProdOutMax=[]  UngainTsProdOutMin=[]  UngainTsProdOutMax=[]  IntegratorContinuousStateAttributes=''  IntegratorStateMustResolveToSignalObject=off  IntegratorRTWStateStorageClass=Auto  FilterContinuousStateAttributes=''  FilterStateMustResolveToSignalObject=off  FilterRTWStateStorageClass=Auto  ParallelPVariant=InternalParameters  IdealPVariant=Disabled  IVariant=InternalParameters  DVariant=InternalParameters  IntegratorVariant=Discrete  SatVariant=Disabled  AWVariant=Passthrough  PCopyVariant=Disabled  TRVariant=Disabled  FdbkBlocksVariant=Forward  IdealPFdbkVariant=Disabled  SatFdbkVariant=Disabled  DerivativeFilterVariant=ForwardEulerFilter  NVariant=InternalParameters  NCopyVariant=Disabled  FilterICVariant=InternalICsFilter  IntegratorICVariant=InternalICs  ExternalResetVariant=Disabled  TRSumVariant=Passthrough  SumFdbkVariant=Disabled  SumVariant=Sum_PID  TsampFilterVariant=InternalTs  TsampNgainVariant=Passthrough  TsampIntegralVariant=Passthrough  ExternalSaturationOutDataTypeStr=Inherit: Same as second input
  cfblk4 : DiscreteTransferFcn
  cfblk5 : DotProduct  InputSameDT=on  OutDataTypeStr=Inherit: Inherit via internal rule
  cfblk6 : Constant  Value=[245848100.749028]  SampleTime=1
  cfblk7 : Constant  Value=[-173524507.011648]  SampleTime=1
  cfblk8 : Constant  Value=[717107234.241658]  SampleTime=1
  cfblk9 : Constant  Value=[-432121976.870338]  SampleTime=1
  cfblk2 : Outport
  cfblk14 : Outport  Port=2
  wires:
  cfblk4/1 -> cfblk5/1
  cfblk8/1 -> cfblk14/1
  cfblk12/1(cfblk2) -> cfblk5/2
  cfblk15/1(cfblk2) -> cfblk3/1
  cfblk12/2(cfblk13) -> cfblk15/1(cfblk1)
  cfblk6/1 -> cfblk11/1(cfblk1)
  cfblk9/1 -> cfblk16/1(cfblk1)
  cfblk11/1(cfblk2) -> cfblk12/1(cfblk1)
  cfblk10/1 -> cfblk15/2(cfblk11)
  cfblk7/1 -> cfblk12/2(cfblk12)
  cfblk3/1 -> cfblk2/1
  cfblk15/2(cfblk12) -> cfblk4/1
  cfblk16/2(cfblk10) -> cfblk11/2(cfblk14)
  cfblk1/1 -> cfblk11/3(cfblk15)
  cfblk13/1 -> cfblk15/Action
  cfblk13/2 -> cfblk16/Action
  cfblk15/3(cfblk13) -> cfblk17/1
  cfblk17/1 -> cfblk11/4(cfblk16)
  cfblk16/1(cfblk2) -> cfblk18/1
  cfblk18/1 -> cfblk13/1

== system sampleModel1/cfblk103/cfblk5/cfblk19/cfblk12 ==
  cfblk1 : Inport
  cfblk5 : Inport  Port=2
  cfblk6 : Inport  Port=3
  cfblk3 : Bias  Bias=[296574898.451171]
  cfblk4 : Constant  Value=[-38391896.641121]  SampleTime=1
  cfblk2 : Outport
  cfblk7 : Outport  Port=2
  cfblk8 : Outport  Port=3
  wires:
  cfblk4/1 -> cfblk8/1
  cfblk1/1 -> cfblk7/1
  cfblk5/1 -> cfblk2/1
  cfblk6/1 -> cfblk3/1

== system sampleModel1/cfblk103/cfblk5/cfblk20/cfblk12 ==
  cfblk1 : Inport
  cfblk10 : Inport  Port=2
  cfblk11 : Inport  Port=3
  cfblk12 : Inport  Port=4
  cfblk13 : Inport  Port=5
  cfblk14 : Inport  Port=6
  Action Port : ActionPort  ActionPortLabel=if(u1 >= 0)
  cfblk3 : PermuteDimensions
  cfblk4 : UnaryMinus
  cfblk5 : UnaryMinus
  cfblk6 : simulink/Math Operations/Slider Gain  gain=1  low=0  high=2
  cfblk7 : Constant  Value=[149067180.347994]  SampleTime=1
  cfblk8 : Constant  Value=[-9135182.419280]  SampleTime=1
  cfblk9 : Constant  Value=[-348004660.056653]  SampleTime=1
  cfblk2 : Outport
  cfblk15 : Outport  Port=2
  wires:
  cfblk1/1 -> cfblk5/1
  cfblk5/1 -> cfblk2/1
  cfblk12/1 -> cfblk15/1
  cfblk14/1 -> cfblk6/1
  cfblk13/1 -> cfblk4/1
  cfblk11/1 -> cfblk3/1

== system sampleModel1/cfblk103/cfblk5/cfblk20/cfblk13 ==
  cfblk1 : Inport
  cfblk10 : Inport  Port=2
  cfblk11 : Inport  Port=3
  Action Port : ActionPort  ActionPortLabel=else
  cfblk13 : Delay
  cfblk3 : DiscreteTransferFcn
  cfblk4 : Polyval  Coefs=[ +2.081618890e-019, -1.441693666e-014, +4.719686976e-010, -8.536869453e-006, +1.621573104e-001, -8.087801117e+001 ]
  cfblk5 : simulink/Math Operations/MinMax Running Resettable  Function=min  vinit=0.0
  cfblk6 : Gain  Gain=[-903637711.978594]
  cfblk7 : Sum  Inputs=|++
  cfblk8 : simulink/Math Operations/MinMax Running Resettable  Function=min  vinit=0.0
  cfblk9 : Constant  Value=[-561668034.891236]  SampleTime=1
  cfblk2 : Outport
  cfblk12 : Outport  Port=2
  wires:
  cfblk9/1 -> cfblk2/1
  cfblk7/1 -> cfblk3/1
  cfblk3/1 -> cfblk6/1
  cfblk4/1 -> cfblk8/1
  cfblk11/1 -> cfblk5/1
  cfblk10/1 -> cfblk8/2, cfblk5/2
  cfblk6/1 -> cfblk12/1
  cfblk5/1 -> cfblk7/1
  cfblk1/1 -> cfblk7/2
  cfblk8/1 -> cfblk13/1
  cfblk13/1 -> cfblk4/1

== system sampleModel1/cfblk103/cfblk5/cfblk20/cfblk9 ==
  cfblk1 : Inport
  cfblk13 : Inport  Port=2
  cfblk14 : Inport  Port=3
  cfblk10 : Constant  Value=[-700782802.734668]  SampleTime=1
  cfblk11 : Constant  Value=[-328067808.662877]  SampleTime=1
  cfblk12 : Constant  Value=[-26521576.747965]  SampleTime=1
  cfblk3 : simulink/Discrete/Tapped Delay  vinit=0.0  samptime=-1  NumDelays=1  DelayOrder=Oldest  includeCurrent=off
  cfblk4 : Abs
  cfblk5 : PermuteDimensions
  cfblk6 : Sum  Inputs=+-
  cfblk7 : simulink/Math Operations/MinMax Running Resettable  Function=min  vinit=0.0
  cfblk8 : Constant  Value=[68285727.888540]  SampleTime=1
  cfblk9 : Constant  Value=[-272107640.918511]  SampleTime=1
  cfblk2 : Outport
  cfblk15 : Outport  Port=2
  cfblk16 : Outport  Port=3
  wires:
  cfblk13/1 -> cfblk3/1
  cfblk12/1 -> cfblk7/1
  cfblk14/1 -> cfblk7/2
  cfblk4/1 -> cfblk16/1
  cfblk9/1 -> cfblk6/1
  cfblk10/1 -> cfblk5/1
  cfblk1/1 -> cfblk2/1
  cfblk3/1 -> cfblk4/1
  cfblk7/1 -> cfblk15/1
  cfblk5/1 -> cfblk6/2
